simulink model "cycletest6"  (R2023a)
settings: Solver=ode1  StartTime=0.0  StopTime=400  FixedStep=0.003  RelTol=1e-3  EnableMultiTasking=on
values from neighbouring files (symbols this model uses):
  Astate = [0, 1; -1, 4]    [setup_lab_hover.m]
  Bstate = [1, 0; 0, 1]    [setup_lab_hover.m]
  Cstate = [1, 0; 0, 1]    [setup_lab_hover.m]
  cycleGain = 0.2    [simulate_hover.m]    (also in temp.m = 1)
  Dstate = [0, 0; 0, 0]    [setup_lab_hover.m]
  Jp = 2*Jeq_prop    (= 0.0552224595625)    [setup_lab_hover.m]    (also in simulate_hover.m)
  Jr = 2*Jeq_prop    (= 0.0552224595625)    [setup_lab_hover.m]    (also in simulate_hover.m)
  kd = 0.5    [simulate_hover.m]
  Kf = 0.1188    [setup_lab_hover.m]    (also in simulate_hover.m)
  L = 7.75*0.0254    (= 0.19685)    [setup_lab_hover.m]    (also in simulate_hover.m = 0.1969)
  r = flexSize(no)    [phaseComp.m]    (also in simulate_hover.m = 0.5)
  skew = 2    [simulate_hover.m]
  V_bias = 12    [setup_lab_hover.m]    (also in simulate_hover.m)
  velMax = 100*60*pi/180    (= 104.71975512)    [simulate_hover.m]
  VMAX_AMP = 24    [setup_lab_hover.m]    (also in simulate_hover.m)
  wcf = 2 * pi * 20    (= 125.663706144)    [setup_lab_hover.m]    (also in simulate_hover.m)
  x0 = x0(:)    [calc_jacob.m]    (also in setup_lab_hover.m = transpose(0.5*[pi/2, pi/6, pi/6, 0, 0, 0]))
  zetaf = 0.6    [setup_lab_hover.m]    (also in simulate_hover.m)
libraries: simulink_extras x1
settings Model: ExtModeTrigDuration=10000  Creator=kille  LastModifiedBy=Jacob
settings SolverCC: AlgebraicLoopSolver=TrustRegion  PositivePriorityOrder=on
settings DataIOCC: ReturnWorkspaceOutputs=off
settings OptimizationCC: LifeSpan=inf
settings DebuggingCC: UnconnectedInputMsg=warning  UnconnectedOutputMsg=warning  UnconnectedLineMsg=warning  ArithmeticOperatorsInVariantConditions=warning
settings ModelReferenceCC: EnableRefExpFcnMdlSchedulingChecks=on
settings SFSimCC: SimUseLocalCustomCode=off  CustomCodeUndefinedFunction=UseInterfaceOnly
settings RTWCC: Description=QUARC Win64 Target  SystemTargetFile=quarc_win64.tlc  TemplateMakefile=quarc_default_tmf  RTWUseLocalCustomCode=off
settings CodeAppCC: StateflowObjectComments=on
settings STFCustomTargetCC: TargetPreCompLibLocation=C:\PROGRA~3\QUARC\lib\2016a\win64\release  UseToolchainInfoCompliant=off  SystemTargetFile=quarc_win64.tlc
settings GRTTargetCC: TargetPreCompLibLocation=C:\PROGRA~3\QUARC\lib\2016a\win64\release  ParMdlRefBuildCompliant=off  CompOptLevelCompliant=off  CombineOutputUpdateFcns=off  MatFileLogging=off  CPPClassGenCompliant=off  GRTInterface=on  UseToolchainInfoCompliant=off  ExtMode=on  ExtModeMexFile=quarc_comm
settings ConfigComp: CovMetricSettings=dswe

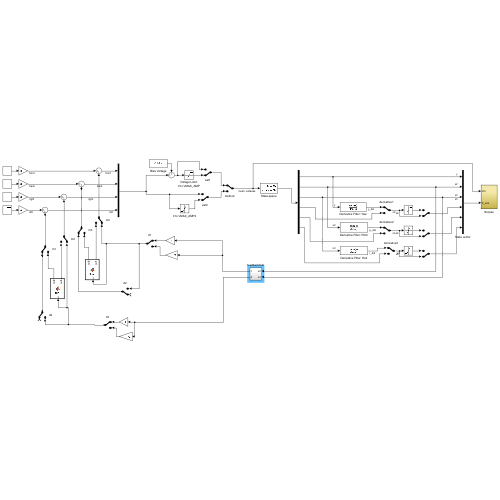
[thumbnail: Simulink's stored preview of the top-level diagram]
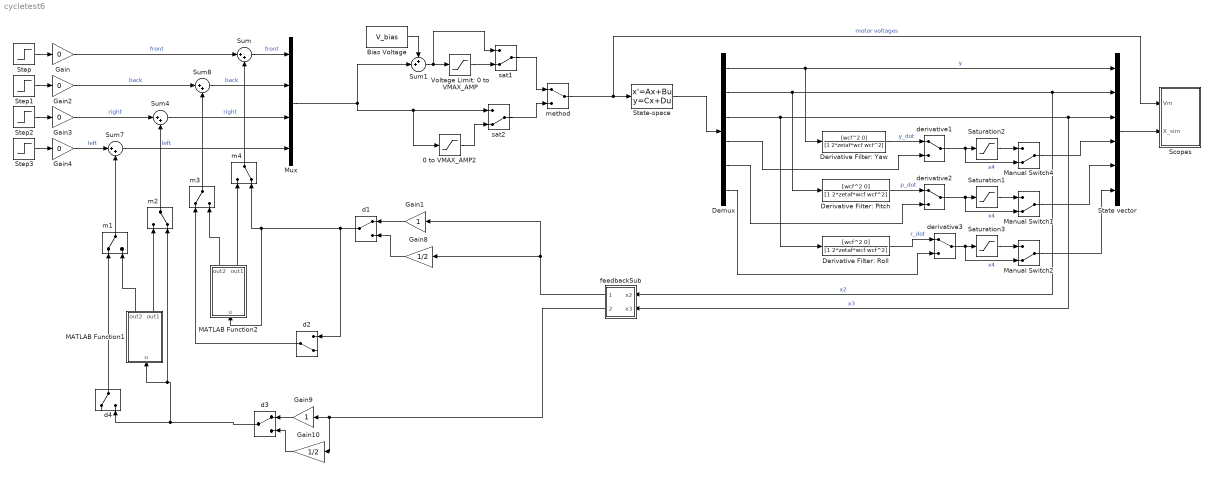
== system cycletest6 ==
  0 to VMAX_AMP2 : Saturate  UpperLimit=VMAX_AMP  LowerLimit=0
  Bias Voltage : Constant  Value=V_bias
  Demux : Demux  Outputs=6
  Derivative Filter: Pitch : TransferFcn  Numerator=[wcf^2 0]  Denominator=[1 2*zetaf*wcf wcf^2]
  Derivative Filter: Roll : TransferFcn  Numerator=[wcf^2 0]  Denominator=[1 2*zetaf*wcf wcf^2]
  Derivative Filter: Yaw : TransferFcn  Numerator=[wcf^2 0]  Denominator=[1 2*zetaf*wcf wcf^2]
  Gain{,2..4} (4 alike) : Gain  Gain=0
  Gain1 : Gain
  Gain10 : Gain  Gain=1/2
  Gain8 : Gain  Gain=1/2
  Gain9 : Gain
  MATLAB Function1 : MATLAB Function  TreatAsAtomicUnit=on
  MATLAB Function2 : MATLAB Function  TreatAsAtomicUnit=on
  Manual Switch1 : ManualSwitch  CurrentSetting=0
  Manual Switch2 : ManualSwitch  CurrentSetting=0
  Manual Switch4 : ManualSwitch  CurrentSetting=0
  Mux : Mux
  Saturation1 : Saturate  UpperLimit=velMax  LowerLimit=-velMax
  Saturation2 : Saturate  UpperLimit=velMax  LowerLimit=-velMax
  Saturation3 : Saturate  UpperLimit=velMax  LowerLimit=-velMax
  Scopes : Subsystem
  State vector : Mux  Inputs=6
  State-space : StateSpace  A=Astate  B=Bstate  C=Cstate  D=Dstate  InitialCondition=x0  ParameterTunability=Unconstrained
  Step{,1..3} (4 alike) : Step  Time=2  Before=-1  After=0  SampleTime=0
  Sum{,4,7..8} (4 alike) : Sum  Inputs=|++
  Sum1 : Sum  Inputs=++|
  Voltage Limit: 0 to VMAX_AMP : Saturate  UpperLimit=VMAX_AMP  LowerLimit=0
  d1 : ManualSwitch
  d2 : ManualSwitch  CurrentSetting=0
  d3 : ManualSwitch
  d4 : ManualSwitch
  derivative1 : ManualSwitch
  derivative2 : ManualSwitch
  derivative3 : ManualSwitch
  feedbackSub : Subsystem
  m1 : ManualSwitch
  m2 : ManualSwitch  CurrentSetting=0
  m3 : ManualSwitch
  m4 : ManualSwitch  CurrentSetting=0
  method : ManualSwitch  Tag=swt
  sat1 : ManualSwitch  CurrentSetting=0
  sat2 : ManualSwitch  CurrentSetting=0
  wires:
  Demux/1 -> State vector/1, Derivative Filter: Yaw/1  "y"
  method/1 -> Scopes/1(Vm), State-space/1  "motor voltages"
  Bias Voltage/1 -> Sum1/1
  State vector/1 -> Scopes/2(X_sim)
  Sum1/1 -> sat1/1, Voltage Limit: 0 to VMAX_AMP/1
  State-space/1 -> Demux/1
  sat1/1 -> method/1
  Voltage Limit: 0 to VMAX_AMP/1 -> sat1/2
  m2/1 -> Sum4/2
  Gain4/1 -> Sum7/1  "left"
  m3/1 -> Sum8/2
  Step3/1 -> Gain4/1
  m4/1 -> Sum/2
  m1/1 -> Sum7/2
  Sum7/1 -> Mux/4  "left"
  Step/1 -> Gain/1
  Gain3/1 -> Sum4/1  "right"
  Gain2/1 -> Sum8/1  "back"
  Sum8/1 -> Mux/2  "back"
  Sum4/1 -> Mux/3  "right"
  Sum/1 -> Mux/1  "front"
  Step1/1 -> Gain2/1
  Step2/1 -> Gain3/1
  Gain/1 -> Sum/1  "front"
  0 to VMAX_AMP2/1 -> sat2/2
  sat2/1 -> method/2
  Mux/1 -> 0 to VMAX_AMP2/1, sat2/1, Sum1/2
  MATLAB Function2/2(out1) -> m4/1
  MATLAB Function2/1(out2) -> m3/2
  MATLAB Function1/2(out1) -> m2/1
  MATLAB Function1/1(out2) -> m1/2
  Derivative Filter: Yaw/1 -> derivative1/1  "y_dot"
  Demux/4 -> derivative1/2
  Derivative Filter: Pitch/1 -> derivative2/1  "p_dot"
  Derivative Filter: Roll/1 -> derivative3/1  "r_dot"
  Demux/5 -> derivative2/2
  Demux/6 -> derivative3/2
  derivative1/1 -> Manual Switch4/2, Saturation2/1  "x4"
  Saturation2/1 -> Manual Switch4/1
  derivative2/1 -> Manual Switch1/2, Saturation1/1  "x4"
  Saturation1/1 -> Manual Switch1/1
  derivative3/1 -> Manual Switch2/2, Saturation3/1  "x4"
  Saturation3/1 -> Manual Switch2/1
  Manual Switch4/1 -> State vector/4
  Manual Switch1/1 -> State vector/5
  Manual Switch2/1 -> State vector/6
  Demux/3 -> State vector/3, feedbackSub/2(x3), Derivative Filter: Roll/1  "x3"
  Demux/2 -> State vector/2, feedbackSub/1(x2), Derivative Filter: Pitch/1  "x2"
  feedbackSub/1(Out1) -> Gain8/1, Gain1/1
  Gain1/1 -> d1/1
  Gain8/1 -> d1/2
  d1/1 -> d2/1, m4/2, MATLAB Function2/1(u)
  d2/1 -> m3/1
  feedbackSub/2(Out2) -> Gain10/1, Gain9/1
  Gain9/1 -> d3/1
  d3/1 -> MATLAB Function1/1(u), m2/2, d4/2
  Gain10/1 -> d3/2
  d4/1 -> m1/1

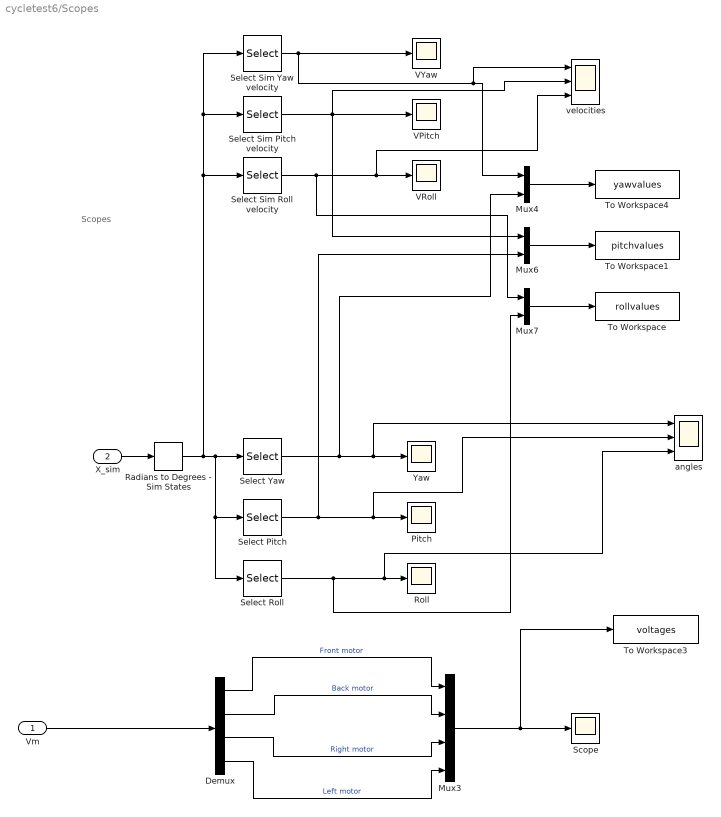
== system cycletest6/Scopes ==
  note: Scopes
  Vm : Inport
  X_sim : Inport  Port=2
  Demux : Demux
  Mux3 : Mux
  Mux4 : Mux  Inputs=2
  Mux6 : Mux  Inputs=2
  Mux7 : Mux  Inputs=2
  Pitch : Scope
  Radians to Degrees - Sim States : simulink_extras/Transformations/Radians to Degrees
  Roll : Scope
  Scope : Scope
  Select Pitch : Selector  InputPortWidth=6  IndexOptions=Index vector (dialog)  Indices=2  OutputSizes=1
  Select Roll : Selector  InputPortWidth=6  IndexOptions=Index vector (dialog)  Indices=3  OutputSizes=1
  Select Sim Pitch velocity : Selector  InputPortWidth=6  IndexOptions=Index vector (dialog)  Indices=5  OutputSizes=1
  Select Sim Roll velocity : Selector  InputPortWidth=6  IndexOptions=Index vector (dialog)  Indices=6  OutputSizes=1
  Select Sim Yaw velocity : Selector  InputPortWidth=6  IndexOptions=Index vector (dialog)  Indices=4  OutputSizes=1
  Select Yaw : Selector  InputPortWidth=6  IndexOptions=Index vector (dialog)  Indices=1  OutputSizes=1
  To Workspace : ToWorkspace  VariableName=rollvalues  SampleTime=-1
  To Workspace1 : ToWorkspace  VariableName=pitchvalues  SampleTime=-1
  To Workspace3 : ToWorkspace  VariableName=voltages  SampleTime=-1
  To Workspace4 : ToWorkspace  VariableName=yawvalues  SampleTime=-1
  VPitch : Scope
  VRoll : Scope
  VYaw : Scope
  Yaw : Scope
  angles : Scope  NumInputPorts=3
  velocities : Scope  NumInputPorts=3
  wires:
  Select Roll/1 -> angles/3, Roll/1, Mux7/2
  Radians to Degrees - Sim States/1 -> Select Sim Roll velocity/1, Select Sim Pitch velocity/1, Select Sim Yaw velocity/1, Select Roll/1, Select Pitch/1, Select Yaw/1
  Select Pitch/1 -> angles/2, Pitch/1, Mux6/2
  X_sim/1 -> Radians to Degrees - Sim States/1
  Demux/1 -> Mux3/1  "Front motor"
  Demux/2 -> Mux3/2  "Back motor"
  Demux/3 -> Mux3/3  "Right motor"
  Demux/4 -> Mux3/4  "Left motor"
  Vm/1 -> Demux/1
  Select Sim Yaw velocity/1 -> VYaw/1, velocities/1, Mux4/1
  Select Sim Roll velocity/1 -> velocities/3, VRoll/1, Mux7/1
  Select Sim Pitch velocity/1 -> Mux6/1, velocities/2, VPitch/1
  Mux4/1 -> To Workspace4/1
  Mux6/1 -> To Workspace1/1
  Mux7/1 -> To Workspace/1
  Mux3/1 -> To Workspace3/1, Scope/1
  Select Yaw/1 -> angles/1, Yaw/1, Mux4/2

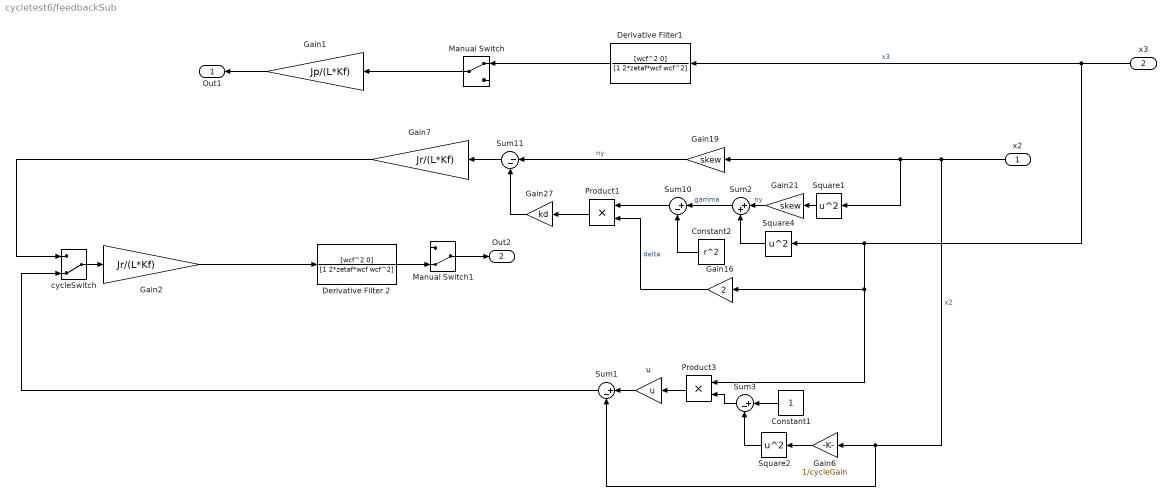
== system cycletest6/feedbackSub ==
  x2 : Inport
  x3 : Inport  Port=2
  Constant1 : Constant
  Constant2 : Constant  Value=r^2
  Derivative Filter 2 : TransferFcn  Numerator=[wcf^2 0]  Denominator=[1 2*zetaf*wcf wcf^2]
  Derivative Filter1 : TransferFcn  Numerator=[wcf^2 0]  Denominator=[1 2*zetaf*wcf wcf^2]
  Gain1 : Gain  Gain=Jp/(L*Kf)
  Gain16 : Gain  Gain=2
  Gain19 : Gain  Gain=skew
  Gain2 : Gain  Gain=Jr/(L*Kf)
  Gain21 : Gain  Gain=skew
  Gain27 : Gain  Gain=kd
  Gain6 : Gain  Gain=1/cycleGain
  Gain7 : Gain  Gain=Jr/(L*Kf)
  Manual Switch : ManualSwitch
  Manual Switch1 : ManualSwitch  CurrentSetting=0
  Product1 : Product
  Product3 : Product
  Square1 : Math  Operator=square
  Square2 : Math  Operator=square
  Square4 : Math  Operator=square
  Sum1 : Sum  Inputs=|+-
  Sum10 : Sum  Inputs=|+-
  Sum11 : Sum  Inputs=|--
  Sum2 : Sum  Inputs=|++
  Sum3 : Sum  Inputs=|+-
  cycleSwitch : ManualSwitch  CurrentSetting=0
  u : Gain  Gain=u
  Out1 : Outport
  Out2 : Outport  Port=2
  wires:
  Square1/1 -> Gain21/1
  Gain1/1 -> Out1/1
  Product1/1 -> Gain27/1
  Square4/1 -> Sum2/2
  Gain19/1 -> Sum11/1  "ny"
  Sum2/1 -> Sum10/1  "gamma"
  Gain16/1 -> Product1/2  "delta"
  Sum10/1 -> Product1/1
  Gain27/1 -> Sum11/2
  Gain21/1 -> Sum2/1  "ny"
  Constant2/1 -> Sum10/2
  Sum11/1 -> Gain7/1
  Sum1/1 -> cycleSwitch/2
  x3/1 -> Derivative Filter1/1, Product3/1, Gain16/1, Square4/1  "x3"
  u/1 -> Sum1/1
  Gain6/1 -> Square2/1
  Product3/1 -> u/1
  Constant1/1 -> Sum3/1
  Sum3/1 -> Product3/2
  Square2/1 -> Sum3/2
  x2/1 -> Gain6/1, Sum1/2, Square1/1, Gain19/1  "x2"
  Gain7/1 -> cycleSwitch/1
  Derivative Filter1/1 -> Manual Switch/1
  Manual Switch/1 -> Gain1/1
  Derivative Filter 2/1 -> Manual Switch1/2
  Manual Switch1/1 -> Out2/1
  cycleSwitch/1 -> Gain2/1
  Gain2/1 -> Derivative Filter 2/1

== matlab function cycletest6/MATLAB Function2 ==
  data: out2 output; u input; out1 output
function [out2, out1] = fcn(u)

if u > 0
    out1 = u;
    out2 = 0;
else
    out1 = 0;
    out2 = -u;
end

== matlab function cycletest6/MATLAB Function1 ==
  data: out2 output; u input; out1 output
function [out2, out1] = fcn(u)

if u > 0
    out1 = u;
    out2 = 0;
else
    out1 = 0;
    out2 = -u;
end
